simulink model "dynamic_withBlock"  (R2023a)
settings: Solver=VariableStepAuto  StartTime=0.0  StopTime=4  RelTol=1e-3
undefined symbols (not defined in the file): ur, urRad
libraries: robotmaniplib x5, robotcorelib x1
settings Model: Creator=ashu  LastModifiedBy=ashu
settings DataIOCC: ReturnWorkspaceOutputs=off

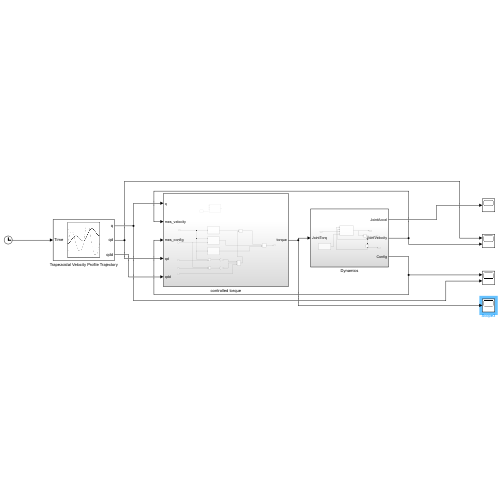
[thumbnail: Simulink's stored preview of the top-level diagram]
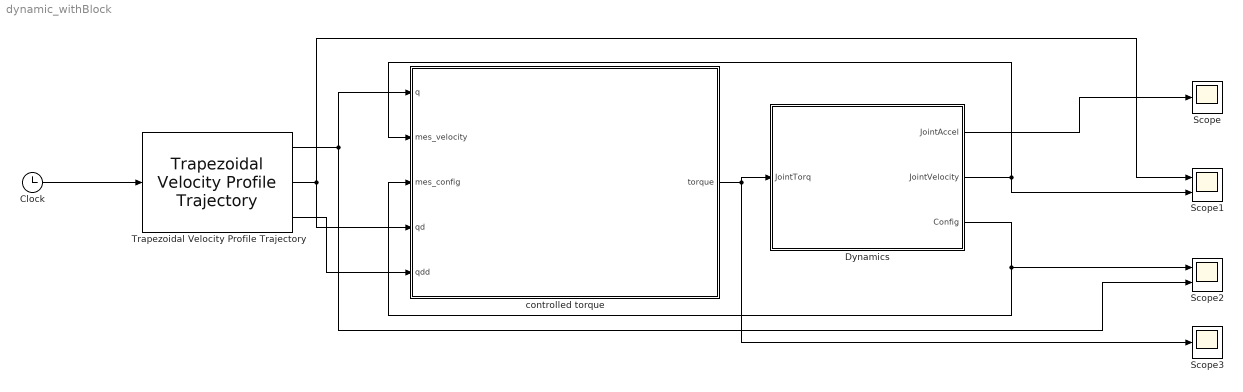
== system dynamic_withBlock ==
  Clock : Clock
  Dynamics : Subsystem
  Scope : Scope
  Scope1 : Scope  NumInputPorts=2
  Scope2 : Scope  NumInputPorts=2
  Scope3 : Scope
  Trapezoidal Velocity Profile Trajectory : robotcorelib/Trapezoidal Velocity Profile Trajectory  WaypointSource=Internal  Waypoints=transpose(urRad)  NumParams=0  Parameter1=Peak Velocity  Parameter2=End Time  ParameterSource=Internal  PeakVelocity=[ 2; 2 ]  Acceleration=[ 1; 2 ]  EndTime=[ 1; 1 ]  AccelTime=[ 1; 2 ]  SimulateUsing=Interpreted execution
  controlled torque : Subsystem
  wires:
  Clock/1 -> Trapezoidal Velocity Profile Trajectory/1
  Trapezoidal Velocity Profile Trajectory/2 -> Scope1/1, controlled torque/4(qd)
  controlled torque/1(torque) -> Scope3/1, Dynamics/1(JointTorq)
  Trapezoidal Velocity Profile Trajectory/1 -> Scope2/2, controlled torque/1(q)
  Trapezoidal Velocity Profile Trajectory/3 -> controlled torque/5(qdd)
  Dynamics/3(Config) -> controlled torque/3(mes_config), Scope2/1
  Dynamics/2(JointVelocity) -> Scope1/2, controlled torque/2(mes_velocity)
  Dynamics/1(JointAccel) -> Scope/1

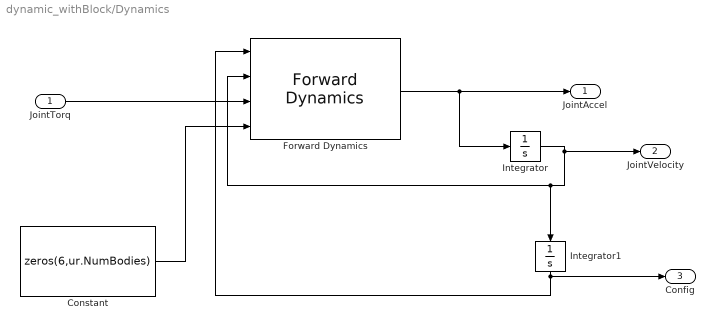
== system dynamic_withBlock/Dynamics ==
  JointTorq : Inport
  Constant : Constant  Value=zeros(6,ur.NumBodies)
  Forward Dynamics : robotmaniplib/Forward Dynamics  RigidBodyTree=ur  SimulateUsing=Interpreted execution
  Integrator : Integrator
  Integrator1 : Integrator
  JointAccel : Outport
  JointVelocity : Outport  Port=2
  Config : Outport  Port=3
  wires:
  JointTorq/1 -> Forward Dynamics/3
  Forward Dynamics/1 -> Integrator/1, JointAccel/1
  Constant/1 -> Forward Dynamics/4
  Integrator/1 -> JointVelocity/1, Forward Dynamics/2, Integrator1/1
  Integrator1/1 -> Forward Dynamics/1, Config/1

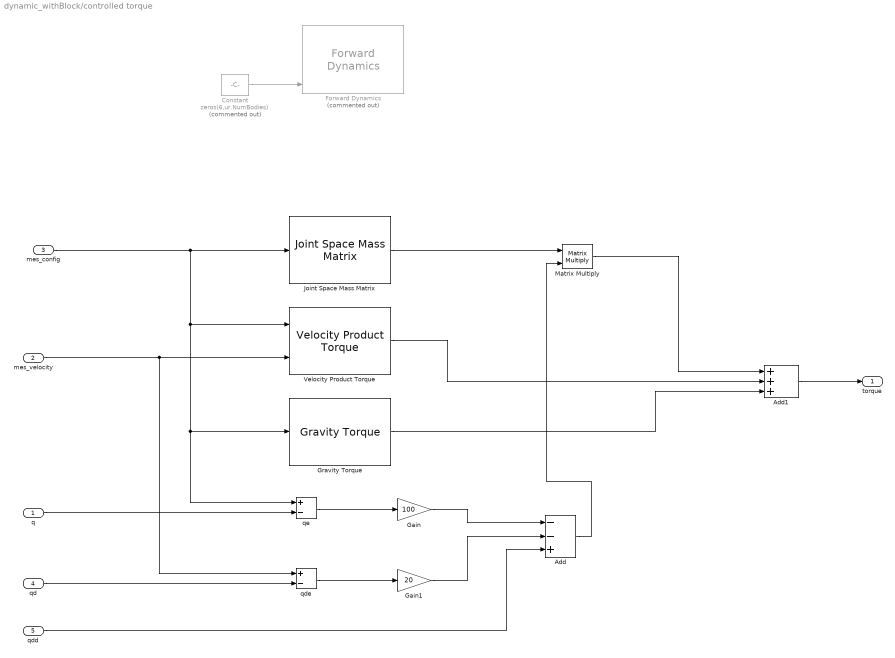
== system dynamic_withBlock/controlled torque ==
  q : Inport
  mes_velocity : Inport  Port=2
  mes_config : Inport  Port=3
  qd : Inport  Port=4
  qdd : Inport  Port=5
  Add : Sum  Inputs=--+
  Add1 : Sum  Inputs=+++
  Constant : Constant  Commented=on  Value=zeros(6,ur.NumBodies)
  Forward Dynamics : robotmaniplib/Forward Dynamics  Commented=on  RigidBodyTree=ur  SimulateUsing=Interpreted execution
  Gain : Gain  Gain=100
  Gain1 : Gain  Gain=20
  Gravity Torque : robotmaniplib/Gravity Torque  RigidBodyTree=ur  SimulateUsing=Interpreted execution
  Joint Space Mass Matrix : robotmaniplib/Joint Space Mass Matrix  RigidBodyTree=ur  SimulateUsing=Interpreted execution
  Matrix Multiply : Product  Multiplication=Matrix(*)
  Velocity Product Torque : robotmaniplib/Velocity Product Torque  RigidBodyTree=ur  SimulateUsing=Interpreted execution
  qde : Sum  Inputs=+-
  qe : Sum  Inputs=+-
  torque : Outport
  wires:
  Add1/1 -> torque/1
  Constant/1 -> Forward Dynamics/4
  qe/1 -> Gain/1
  qde/1 -> Gain1/1
  Gain1/1 -> Add/2
  Gain/1 -> Add/1
  Joint Space Mass Matrix/1 -> Matrix Multiply/1
  Matrix Multiply/1 -> Add1/1
  Velocity Product Torque/1 -> Add1/2
  Gravity Torque/1 -> Add1/3
  Add/1 -> Matrix Multiply/2
  mes_config/1 -> qe/1, Gravity Torque/1, Velocity Product Torque/1, Joint Space Mass Matrix/1
  mes_velocity/1 -> qde/1, Velocity Product Torque/2
  q/1 -> qe/2
  qd/1 -> qde/2
  qdd/1 -> Add/3
